simulink model "Simulator_DecMPC_v0"  (R2023a)
settings: Solver=ode45  StartTime=0  StopTime=50000  RelTol=1e-3
values from neighbouring files (symbols this model uses):
  A = Household_DecMPC(T_set, T_amb, Ts, K, Q)    [main.m]    (also in mainDecMPC.m = Household_DecMPC(T_set, T_amb, Ts, K, Q, 'Simulator_DecMPC_v; mainDecMPC_v1.m = Household_DecMPC(T_set, T_amb, Ts, K,[NAME_SIMULATION '/' AD)
  B = Household_DecMPC(T_set, T_amb, Ts, K, Q)    [main.m]    (also in mainDecMPC_v1.m = Household_DecMPC(T_set, T_amb, Ts, K, [NAME_SIMULATION '/' A)
  C = Household_DecMPC(T_set, T_amb, Ts, K, Q)    [main.m]    (also in mainDecMPC_v1.m = Household_DecMPC(T_set, T_amb, Ts, K, [NAME_SIMULATION '/' A)
  K = 10    [main.m]    (also in mainDecMPC.m; mainDecMPC_v1.m = 4)
  T_set = 350    [main.m]    (also in mainDecMPC.m; mainDecMPC_v1.m = 291)
libraries: mpclib x3
settings Model: Creator=alex  LastModifiedBy=giaco

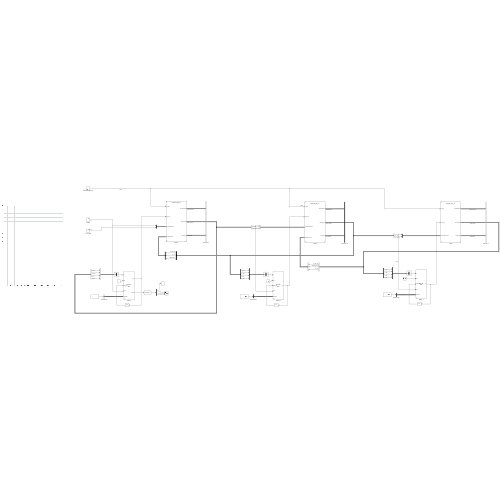
[thumbnail: Simulink's stored preview of the top-level diagram]
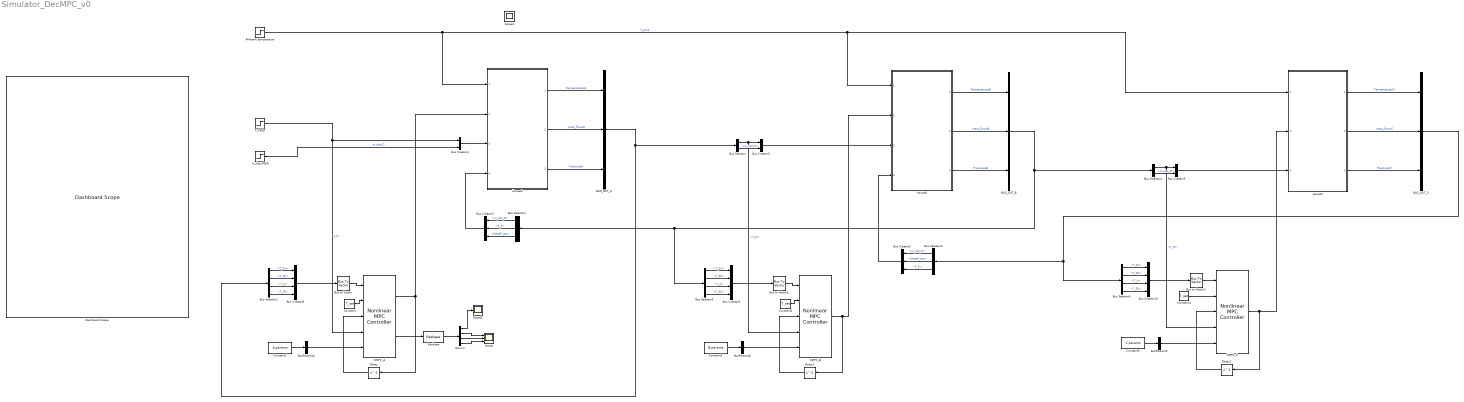
== system Simulator_DecMPC_v0 ==
  Ambient temperature : Step  Time=0  Before=300  After=300  SampleTime=0
  BUS_OUT_A : BusCreator  Inputs=3
  BUS_OUT_B : BusCreator  Inputs=3
  BUS_OUT_C : BusCreator  Inputs=3
  Bus Creator10 : BusCreator  Inputs=4
  Bus Creator2 : BusCreator  Inputs=3
  Bus Creator3 : BusCreator  Inputs=2
  Bus Creator4 : BusCreator  Inputs=2
  Bus Creator5 : BusCreator  Inputs=2
  Bus Creator6 : BusCreator  Inputs=3
  Bus Creator8 : BusCreator  Inputs=4
  Bus Creator9 : BusCreator  Inputs=4
  Bus Selector : BusSelector  OutputSignals=TemperaturesA.T_O,mass_flowsA.m_dot_O
  Bus Selector1 : BusSelector  OutputSignals=mass_flowsB.m_dot_R,TemperaturesB.T_R,PressuresB.DeltaP_tot
  Bus Selector2 : BusSelector  OutputSignals=TemperaturesA.T_S1,TemperaturesA.T_S2,TemperaturesA.T_b,TemperaturesA.T_S3
  Bus Selector3 : BusSelector  OutputSignals=TemperaturesB.T_S1,TemperaturesB.T_S2,TemperaturesB.T_b,TemperaturesB.T_S3
  Bus Selector4 : BusSelector  OutputSignals=TemperaturesB.T_O,mass_flowsB.m_dot_O
  Bus Selector5 : BusSelector  OutputSignals=TemperaturesC.T_S1,TemperaturesC.T_S2,TemperaturesC.T_b,TemperaturesC.T_S3
  Bus Selector6 : BusSelector  OutputSignals=mass_flowsC.m_dot_R,PressuresC.DeltaP_tot,TemperaturesC.T_R
  Bus to Vector : BusToVector
  Bus to Vector1 : BusToVector
  Bus to Vector2 : BusToVector
  BusParamsA : BusCreator  Inputs=1  OutDataTypeStr=Bus: BusParamsC  NonVirtualBus=on
      settings: InheritFromInputs=off
  BusParamsB : BusCreator  Inputs=1  OutDataTypeStr=Bus: BusParamsA  NonVirtualBus=on
      settings: InheritFromInputs=off
  BusParamsC : BusCreator  Inputs=1  OutDataTypeStr=Bus: BusParamsA  NonVirtualBus=on
      settings: InheritFromInputs=off
  Constant : Constant  Value=T_set
  Constant1 : Constant  Value=A.params
  Constant2 : Constant  Value=T_set
  Constant3 : Constant  Value=B.params
  Constant4 : Constant  Value=T_set
  Constant5 : Constant  Value=C.params
  Dashboard Scope : DashboardScope
  Delay : Delay  DelayLength=1
  Delay1 : Delay  DelayLength=1
  Delay2 : Delay  DelayLength=1
  Demux : Demux
  HouseA : Subsystem  ReferencedSubsystem=Simulator_MID_v4  rho=971  c_p=4179  pi=3.14151  f_Darcy=0.025  L_F=40.5  D_F=0.4  h_F=1.5  D_S1=1  L_S1=0.4  h_S1=1.5  D_S2=0.4  L_S2=50  h_S2=1.5  D_S3=0.4  L_S3=5  h_S3=1.5  D_R=0.4  L_R=40  h_R=1.5  C_b=300  A_b=500  h_b=1.5  T_F_0=273  T_S1_0=273  T_S2_0=273  T_S3_0=273  T_b_0=273  T_R_0=273
  HouseB : Subsystem  ReferencedSubsystem=Simulator_MID_v4  rho=971  c_p=4179  pi=3.14151  f_Darcy=0.025  L_F=40.5  D_F=0.4  h_F=1.5  D_S1=1  L_S1=0.4  h_S1=1.5  D_S2=0.4  L_S2=50  h_S2=1.5  D_S3=0.4  L_S3=5  h_S3=1.5  D_R=0.4  L_R=40  h_R=1.5  C_b=300  A_b=500  h_b=1.5  T_F_0=273  T_S1_0=273  T_S2_0=273  T_S3_0=273  T_b_0=273  T_R_0=273
  HouseC : Subsystem  ReferencedSubsystem=Simulator_BYP_v4  rho=971  rho_air=971  c_p=4179  c_p_air=4179  pi=3.14151  f_Darcy=0.025  L_F=40.5  D_F=0.4  h_F=1.5  D_S1=0.4  L_S1=5  h_S1=1.5  D_S2=0.4  L_S2=5000  h_S2=300  D_S3=0.4  L_S3=5  h_S3=0.4  D_R=0.4  L_R=40  h_R=1.5  C_b=100  A_b=500  h_b=1.5  D_BYP=0.1  L_BYP=3  h_BYP=1.5  T_F_0=273  T_S1_0=273  T_S2_0=273  T_S3_0=273  T_b_0=273  T_R_0=273
  NMPC_A : mpclib/Nonlinear MPC Controller  nlmpcobj=A.nlobj  UseObjectTs=on  UseMEX=off  md_enabled=on  mvtarget_enabled=off  param_enabled=on  cost_enabled=off  mvseq_enabled=off  stateseq_enabled=on  ovseq_enabled=off  slack_enabled=off  status_enabled=off  ov_min=off  ov_max=off  mv_min=off  mv_max=off  mvrate_min=off  mvrate_max=off  state_min=off  state_max=off  ov_weight=off  mv_weight=off  mvrate_weight=off  ecr_weight=off  nlp_initialize=off
  NMPC_B : mpclib/Nonlinear MPC Controller  nlmpcobj=A.nlobj  UseObjectTs=on  UseMEX=off  md_enabled=on  mvtarget_enabled=off  param_enabled=on  cost_enabled=off  mvseq_enabled=off  stateseq_enabled=off  ovseq_enabled=off  slack_enabled=off  status_enabled=off  ov_min=off  ov_max=off  mv_min=off  mv_max=off  mvrate_min=off  mvrate_max=off  state_min=off  state_max=off  ov_weight=off  mv_weight=off  mvrate_weight=off  ecr_weight=off  nlp_initialize=off
  NMPC_C : mpclib/Nonlinear MPC Controller  nlmpcobj=A.nlobj  UseObjectTs=on  UseMEX=off  md_enabled=on  mvtarget_enabled=off  param_enabled=on  cost_enabled=off  mvseq_enabled=off  stateseq_enabled=off  ovseq_enabled=off  slack_enabled=off  status_enabled=off  ov_min=off  ov_max=off  mv_min=off  mv_max=off  mvrate_min=off  mvrate_max=off  state_min=off  state_max=off  ov_weight=off  mv_weight=off  mvrate_weight=off  ecr_weight=off  nlp_initialize=off
  Reshape : Reshape  OutputDimensionality=Customize  OutputDimensions=[(K+1)*4,1]
  Scope : Scope  NumInputPorts=3
  Scope2 : Scope
  T_FEED : Step  Time=0  After=350  SampleTime=0
  m_dot_FEED : Step  Time=0  Before=15  After=10000  SampleTime=0
  Scope1 : Scope
  wires:
  HouseA/1 -> BUS_OUT_A/1  "TemperaturesA"
  HouseA/2 -> BUS_OUT_A/2  "mass_flowsA"
  HouseA/3 -> BUS_OUT_A/3  "PressuresA"
  Ambient temperature/1 -> HouseA/1, HouseC/1, HouseB/1  "T_amb"
  HouseB/1 -> BUS_OUT_B/1  "TemperaturesB"
  HouseB/2 -> BUS_OUT_B/2  "mass_flowsB"
  HouseB/3 -> BUS_OUT_B/3  "PressuresB"
  Bus Selector1/1 -> Bus Creator2/1  "<m_dot_R>"
  Bus Selector1/2 -> Bus Creator2/2  "<T_R>"
  Bus Selector1/3 -> Bus Creator2/3  "<DeltaP_tot>"
  Bus Creator2/1 -> HouseA/4
  Bus Creator3/1 -> HouseB/3
  BUS_OUT_A/1 -> Bus Selector/1, Bus Selector2/1
  Bus Selector/2 -> Bus Creator3/2  "<m_dot_O>"
  Bus Creator4/1 -> HouseA/3
  Bus Selector4/2 -> Bus Creator5/2  "<m_dot_O>"
  Bus Creator5/1 -> HouseC/3
  Bus Creator6/1 -> HouseB/4
  Bus Selector6/3 -> Bus Creator6/3  "<T_R>"
  Bus Selector6/2 -> Bus Creator6/2  "<DeltaP_tot>"
  Bus Selector6/1 -> Bus Creator6/1  "<m_dot_R>"
  HouseC/3 -> BUS_OUT_C/3  "PressuresC"
  HouseC/2 -> BUS_OUT_C/2  "mass_flowsC"
  HouseC/1 -> BUS_OUT_C/1  "TemperaturesC"
  NMPC_C/1 -> HouseC/2, Delay2/1
  T_FEED/1 -> Bus Creator4/1, NMPC_A/4  "T_O"
  m_dot_FEED/1 -> Bus Creator4/2  "m_dot_O"
  NMPC_A/1 -> Delay/1, HouseA/2
  Bus Selector2/1 -> Bus Creator8/1  "<T_S1>"
  Bus Selector2/2 -> Bus Creator8/2  "<T_S2>"
  Bus Selector2/3 -> Bus Creator8/3  "<T_b>"
  Bus Selector2/4 -> Bus Creator8/4  "<T_S3>"
  Bus Creator8/1 -> Bus to Vector/1
  Bus to Vector/1 -> NMPC_A/1
  Delay/1 -> NMPC_A/3
  Constant/1 -> NMPC_A/2
  BusParamsA/1 -> NMPC_A/5
  Constant1/1 -> BusParamsA/1
  BUS_OUT_B/1 -> Bus Selector4/1, Bus Selector3/1, Bus Selector1/1
  Bus Selector3/2 -> Bus Creator9/2  "<T_S2>"
  Bus Selector3/4 -> Bus Creator9/4  "<T_S3>"
  Bus Selector3/1 -> Bus Creator9/1  "<T_S1>"
  NMPC_B/1 -> HouseB/2, Delay1/1
  BusParamsB/1 -> NMPC_B/5
  Bus Selector3/3 -> Bus Creator9/3  "<T_b>"
  Bus Creator9/1 -> Bus to Vector1/1
  Constant2/1 -> NMPC_B/2
  Delay1/1 -> NMPC_B/3
  Bus to Vector1/1 -> NMPC_B/1
  Bus Selector/1 -> Bus Creator3/1, NMPC_B/4  "<T_O>"
  Constant3/1 -> BusParamsB/1
  Bus to Vector2/1 -> NMPC_C/1
  Bus Selector5/2 -> Bus Creator10/2  "<T_S2>"
  BusParamsC/1 -> NMPC_C/5
  Bus Selector5/4 -> Bus Creator10/4  "<T_S3>"
  Bus Selector5/3 -> Bus Creator10/3  "<T_b>"
  Bus Creator10/1 -> Bus to Vector2/1
  Constant4/1 -> NMPC_C/2
  Delay2/1 -> NMPC_C/3
  Bus Selector5/1 -> Bus Creator10/1  "<T_S1>"
  Constant5/1 -> BusParamsC/1
  BUS_OUT_C/1 -> Bus Selector6/1, Bus Selector5/1
  Bus Selector4/1 -> NMPC_C/4, Bus Creator5/1  "<T_O>"
  NMPC_A/2 -> Reshape/1
  Demux/1 -> Scope2/1
  Demux/2 -> Scope/1
  Demux/3 -> Scope/2
  Demux/4 -> Scope/3
  Reshape/1 -> Demux/1
